simulink model "s_c856m4k_cd"  (R2016b)
settings: Solver=VariableStepAuto  StartTime=0.0  StopTime=3000  RelTol=1e-3  EnableMultiTasking=on
undefined symbols (not defined in the file): fft_stages
libraries: xbsIndex_r4 x8343, casper_library_misc x49, casper_library_scopes x9, xps_library x1, casper_library_communications x1
(part 18 of 60)

== system s_c856m4k_cd/cd_compensation0/cd_hmc/delay_wideband_prog ==
  sync : Inport
  delay : Inport  Port=2
  ld_delay : Inport  Port=3
  data_in0 : Inport  Port=4
  data_in1 : Inport  Port=5
  data_in2 : Inport  Port=6
  data_in3 : Inport  Port=7
  data_in4 : Inport  Port=8
  data_in5 : Inport  Port=9
  data_in6 : Inport  Port=10
  data_in7 : Inport  Port=11
  en : Inport  Port=12
  AddSub{1..7} (7 alike) : xbsIndex_r4/AddSub  mode=Addition  use_carryin=off  use_carryout=off  en=off  latency=0  precision=Full  arith_type=Unsigned  n_bits=1  bin_pt=0  quantization=Truncate  overflow=Wrap  use_behavioral_HDL=off  hw_selection=Fabric  pipelined=off  dbl_ovrd=off  block_type=addsub
  Constant1 : xbsIndex_r4/Constant  const=6  gui_display_data_type=Fixed-point  arith_type=Unsigned  n_bits=3  bin_pt=0  preci_type=Single  exp_width=8  frac_width=24  explicit_period=on  period=1  equ=P=C  opselect=C  inp2=PCIN>>17  opr=+  inp1=P  carry=CIN  dbl_ovrd=off  block_type=constant
  Constant2 : xbsIndex_r4/Constant  const=5  gui_display_data_type=Fixed-point  arith_type=Unsigned  n_bits=3  bin_pt=0  preci_type=Single  exp_width=8  frac_width=24  explicit_period=on  period=1  equ=P=C  opselect=C  inp2=PCIN>>17  opr=+  inp1=P  carry=CIN  dbl_ovrd=off  block_type=constant
  Constant3 : xbsIndex_r4/Constant  const=4  gui_display_data_type=Fixed-point  arith_type=Unsigned  n_bits=3  bin_pt=0  preci_type=Single  exp_width=8  frac_width=24  explicit_period=on  period=1  equ=P=C  opselect=C  inp2=PCIN>>17  opr=+  inp1=P  carry=CIN  dbl_ovrd=off  block_type=constant
  Constant4 : xbsIndex_r4/Constant  const=3  gui_display_data_type=Fixed-point  arith_type=Unsigned  n_bits=3  bin_pt=0  preci_type=Single  exp_width=8  frac_width=24  explicit_period=on  period=1  equ=P=C  opselect=C  inp2=PCIN>>17  opr=+  inp1=P  carry=CIN  dbl_ovrd=off  block_type=constant
  Constant5 : xbsIndex_r4/Constant  const=2  gui_display_data_type=Fixed-point  arith_type=Unsigned  n_bits=3  bin_pt=0  preci_type=Single  exp_width=8  frac_width=24  explicit_period=on  period=1  equ=P=C  opselect=C  inp2=PCIN>>17  opr=+  inp1=P  carry=CIN  dbl_ovrd=off  block_type=constant
  Constant6 : xbsIndex_r4/Constant  const=1  gui_display_data_type=Fixed-point  arith_type=Unsigned  n_bits=3  bin_pt=0  preci_type=Single  exp_width=8  frac_width=24  explicit_period=on  period=1  equ=P=C  opselect=C  inp2=PCIN>>17  opr=+  inp1=P  carry=CIN  dbl_ovrd=off  block_type=constant
  Constant7 : xbsIndex_r4/Constant  const=0  gui_display_data_type=Fixed-point  arith_type=Unsigned  n_bits=3  bin_pt=0  preci_type=Single  exp_width=8  frac_width=24  explicit_period=on  period=1  equ=P=C  opselect=C  inp2=PCIN>>17  opr=+  inp1=P  carry=CIN  dbl_ovrd=off  block_type=constant
  Convert{1..7} (7 alike) : xbsIndex_r4/Convert  gui_display_data_type=Fixed-point  arith_type=Unsigned  n_bits=1  bin_pt=0  float_type=Single  exp_bits=8  fraction_bits=24  quantization=Truncate  overflow=Wrap  en=off  latency=0  pipeline=off  dbl_ovrd=off  block_type=convert
  Relational{1..7} (7 alike) : xbsIndex_r4/Relational  mode=a>b  op_type=Bool  en=off  latency=0  dbl_ovrd=off  block_type=relational
  barrel_switcher : Subsystem  AncestorBlock=casper_library_reorder/barrel_switcher  mask(barrel_switcher){n_inputs=3, async=on}
      mask prompts: n_inputs "Number of Inputs: (2^?)"; async "Asynchronous operation"
      mask help:
      | Shifts input to right by amount specified on sel,
      | wrapping around into higher order bits.
      mask init:
      | barrel_switcher_init(gcb,...
      |     'n_inputs', n_inputs, ...
      |     'async', async);
      mask Help: eval('xlWeb(''http://casper.berkeley.edu/wiki/Barrel_switcher'')')
  bram_rd_addrs : xbsIndex_r4/Slice  nbits=1  boolean_output=off  mode=Lower Bit Location + Width  bit1=0  base1=MSB of Input  bit0=3  base0=LSB of Input  dbl_ovrd=off  block_type=slice
  delay_dp0 : Subsystem  AncestorBlock=casper_library_delays/delay_bram_prog_dp  mask(delay_bram_prog_dp){ram_bits=2, bram_latency=3, async=on}
      mask prompts: ram_bits "Max delay (2^?)"; bram_latency "BRAM latency"; async "asynchronous operation"
      mask init:
      | %delay_bram_prog_dp_init(gcb, ...
      | %    'ram_bits', ram_bits, ...
      | %    'bram_latency', bram_latency, ...
      | %    'async', async);
  delay_dp1 : Subsystem  AncestorBlock=casper_library_delays/delay_bram_prog_dp  mask(delay_bram_prog_dp){ram_bits=2, bram_latency=3, async=on}
      mask prompts: ram_bits "Max delay (2^?)"; bram_latency "BRAM latency"; async "asynchronous operation"
      mask init:
      | %delay_bram_prog_dp_init(gcb, ...
      | %    'ram_bits', ram_bits, ...
      | %    'bram_latency', bram_latency, ...
      | %    'async', async);
  delay_dp2 : Subsystem  AncestorBlock=casper_library_delays/delay_bram_prog_dp  mask(delay_bram_prog_dp){ram_bits=2, bram_latency=3, async=on}
      mask prompts: ram_bits "Max delay (2^?)"; bram_latency "BRAM latency"; async "asynchronous operation"
      mask init:
      | %delay_bram_prog_dp_init(gcb, ...
      | %    'ram_bits', ram_bits, ...
      | %    'bram_latency', bram_latency, ...
      | %    'async', async);
  delay_dp3 : Subsystem  AncestorBlock=casper_library_delays/delay_bram_prog_dp  mask(delay_bram_prog_dp){ram_bits=2, bram_latency=3, async=on}
      mask prompts: ram_bits "Max delay (2^?)"; bram_latency "BRAM latency"; async "asynchronous operation"
      mask init:
      | %delay_bram_prog_dp_init(gcb, ...
      | %    'ram_bits', ram_bits, ...
      | %    'bram_latency', bram_latency, ...
      | %    'async', async);
  delay_dp4 : Subsystem  AncestorBlock=casper_library_delays/delay_bram_prog_dp  mask(delay_bram_prog_dp){ram_bits=2, bram_latency=3, async=on}
      mask prompts: ram_bits "Max delay (2^?)"; bram_latency "BRAM latency"; async "asynchronous operation"
      mask init:
      | %delay_bram_prog_dp_init(gcb, ...
      | %    'ram_bits', ram_bits, ...
      | %    'bram_latency', bram_latency, ...
      | %    'async', async);
  delay_dp5 : Subsystem  AncestorBlock=casper_library_delays/delay_bram_prog_dp  mask(delay_bram_prog_dp){ram_bits=2, bram_latency=3, async=on}
      mask prompts: ram_bits "Max delay (2^?)"; bram_latency "BRAM latency"; async "asynchronous operation"
      mask init:
      | %delay_bram_prog_dp_init(gcb, ...
      | %    'ram_bits', ram_bits, ...
      | %    'bram_latency', bram_latency, ...
      | %    'async', async);
  delay_dp6 : Subsystem  AncestorBlock=casper_library_delays/delay_bram_prog_dp  mask(delay_bram_prog_dp){ram_bits=2, bram_latency=3, async=on}
      mask prompts: ram_bits "Max delay (2^?)"; bram_latency "BRAM latency"; async "asynchronous operation"
      mask init:
      | %delay_bram_prog_dp_init(gcb, ...
      | %    'ram_bits', ram_bits, ...
      | %    'bram_latency', bram_latency, ...
      | %    'async', async);
  delay_dp7 : Subsystem  AncestorBlock=casper_library_delays/delay_bram_prog_dp  mask(delay_bram_prog_dp){ram_bits=2, bram_latency=3, async=on}
      mask prompts: ram_bits "Max delay (2^?)"; bram_latency "BRAM latency"; async "asynchronous operation"
      mask init:
      | %delay_bram_prog_dp_init(gcb, ...
      | %    'ram_bits', ram_bits, ...
      | %    'bram_latency', bram_latency, ...
      | %    'async', async);
  delay_reg : xbsIndex_r4/Register  init=0  rst=off  en=on  dbl_ovrd=off  block_type=register
  delay_sel : xbsIndex_r4/Delay  rst=off  infoeditControl=Selection of Reset will increase slice count due to use of real FFs and instead of SRLs  en=off  latency=4  reg_retiming=on  dbl_ovrd=off  block_type=delay
  en_delay0 : xbsIndex_r4/Delay  rst=off  infoeditControl=Selection of Reset will increase slice count due to use of real FFs and instead of SRLs  en=off  latency=0  reg_retiming=on  dbl_ovrd=off  block_type=delay
  en_delay1 : xbsIndex_r4/Delay  rst=off  infoeditControl=Selection of Reset will increase slice count due to use of real FFs and instead of SRLs  en=off  latency=4  reg_retiming=on  dbl_ovrd=off  block_type=delay
  shift_sel : xbsIndex_r4/Slice  nbits=3  boolean_output=off  mode=Lower Bit Location + Width  bit1=0  base1=MSB of Input  bit0=0  base0=LSB of Input  dbl_ovrd=off  block_type=slice
  sync_delay : xbsIndex_r4/Delay  rst=off  infoeditControl=Selection of Reset will increase slice count due to use of real FFs and instead of SRLs  en=off  latency=4  reg_retiming=on  dbl_ovrd=off  block_type=delay
  sync_out : Outport
  data_out0 : Outport  Port=2
  data_out1 : Outport  Port=3
  data_out2 : Outport  Port=4
  data_out3 : Outport  Port=5
  data_out4 : Outport  Port=6
  data_out5 : Outport  Port=7
  data_out6 : Outport  Port=8
  data_out7 : Outport  Port=9
  dvalid : Outport  Port=10
  wires:
  en/1 -> en_delay0/1
  en_delay0/1 -> en_delay1/1, delay_dp0/3(en), delay_dp1/3(en), delay_dp2/3(en), delay_dp3/3(en), delay_dp4/3(en), delay_dp5/3(en), delay_dp6/3(en), delay_dp7/3(en)  "dp_en"
  sync/1 -> sync_delay/1
  delay/1 -> delay_reg/1
  ld_delay/1 -> delay_reg/2
  delay_reg/1 -> bram_rd_addrs/1, shift_sel/1
  sync_delay/1 -> barrel_switcher/2(sync_in)
  barrel_switcher/1(sync_out) -> sync_out/1
  en_delay1/1 -> barrel_switcher/11(en)
  barrel_switcher/10(dvalid) -> dvalid/1
  shift_sel/1 -> delay_sel/1, Relational1/1, Relational2/1, Relational3/1, Relational4/1, Relational5/1, Relational6/1, Relational7/1
  delay_sel/1 -> barrel_switcher/1(sel)
  barrel_switcher/9(Out8) -> data_out0/1
  barrel_switcher/8(Out7) -> data_out1/1
  barrel_switcher/7(Out6) -> data_out2/1
  barrel_switcher/6(Out5) -> data_out3/1
  barrel_switcher/5(Out4) -> data_out4/1
  barrel_switcher/4(Out3) -> data_out5/1
  barrel_switcher/3(Out2) -> data_out6/1
  barrel_switcher/2(Out1) -> data_out7/1
  data_in0/1 -> delay_dp0/1(din)  "dp_val0"
  delay_dp0/1(dout) -> barrel_switcher/10(In8)
  bram_rd_addrs/1 -> delay_dp0/2(delay), AddSub1/1, AddSub2/1, AddSub3/1, AddSub4/1, AddSub5/1, AddSub6/1, AddSub7/1  "dp0"
  data_in1/1 -> delay_dp1/1(din)  "dp_val1"
  delay_dp1/1(dout) -> barrel_switcher/9(In7)
  Constant1/1 -> Relational1/2
  Relational1/1 -> Convert1/1
  Convert1/1 -> AddSub1/2
  AddSub1/1 -> delay_dp1/2(delay)  "dp1"
  data_in2/1 -> delay_dp2/1(din)  "dp_val2"
  delay_dp2/1(dout) -> barrel_switcher/8(In6)
  Constant2/1 -> Relational2/2
  Relational2/1 -> Convert2/1
  Convert2/1 -> AddSub2/2
  AddSub2/1 -> delay_dp2/2(delay)  "dp2"
  data_in3/1 -> delay_dp3/1(din)  "dp_val3"
  delay_dp3/1(dout) -> barrel_switcher/7(In5)
  Constant3/1 -> Relational3/2
  Relational3/1 -> Convert3/1
  Convert3/1 -> AddSub3/2
  AddSub3/1 -> delay_dp3/2(delay)  "dp3"
  data_in4/1 -> delay_dp4/1(din)  "dp_val4"
  delay_dp4/1(dout) -> barrel_switcher/6(In4)
  Constant4/1 -> Relational4/2
  Relational4/1 -> Convert4/1
  Convert4/1 -> AddSub4/2
  AddSub4/1 -> delay_dp4/2(delay)  "dp4"
  data_in5/1 -> delay_dp5/1(din)  "dp_val5"
  delay_dp5/1(dout) -> barrel_switcher/5(In3)
  Constant5/1 -> Relational5/2
  Relational5/1 -> Convert5/1
  Convert5/1 -> AddSub5/2
  AddSub5/1 -> delay_dp5/2(delay)  "dp5"
  data_in6/1 -> delay_dp6/1(din)  "dp_val6"
  delay_dp6/1(dout) -> barrel_switcher/4(In2)
  Constant6/1 -> Relational6/2
  Relational6/1 -> Convert6/1
  Convert6/1 -> AddSub6/2
  AddSub6/1 -> delay_dp6/2(delay)  "dp6"
  data_in7/1 -> delay_dp7/1(din)  "dp_val7"
  delay_dp7/1(dout) -> barrel_switcher/3(In1)
  Constant7/1 -> Relational7/2
  Relational7/1 -> Convert7/1
  Convert7/1 -> AddSub7/2
  AddSub7/1 -> delay_dp7/2(delay)  "dp7"
